simulink model "my_dspsdadc_fixpt"  (Simulink 7.5)
settings: Solver=ode5  SolverMode=SingleTasking  StartTime=0.0  StopTime=.025  FixedStep=1/(512*1024)  MaxStep=1/512000  RelTol=1e-3  AbsTol=1e-6
values from neighbouring files (symbols this model uses):
  Fs = 100000    [bandwidth_chop.m]
undefined symbols (not defined in the file or in its folder): get, sided, Two
libraries: simulink x42, dspsigops x6, dspsnks4 x2, dsparch4 x1, dspmlti4 x1, dspmisc x1
settings Model: Creator=The MathWorks Inc.  LastModifiedBy=Ben  ExtModeTrigMode=oneshot  ExtModeArmWhenConnect=off  ExtModeAutoUpdateStatusClock=off
settings DataIOCC: LimitDataPoints=off  SaveOutput=off  SaveTime=off  SignalLoggingName=logsOut
settings OptimizationCC: BlockReduction=off  BooleanDataType=off  InlineInvariantSignals=on  RollThreshold=2  InitFltsAndDblsToZero=on  EfficientMapNaN2IntZero=off
settings DebuggingCC: SaveWithParameterizedLinksMsg=none  SignalResolutionControl=TryResolveAllWithWarning  SolverPrmCheckMsg=none  MultiTaskDSMMsg=warning  MultiTaskCondExecSysMsg=none  IntegerOverflowMsg=none  ParameterPrecisionLossMsg=none  StrictBusMsg=None  LoggingUnavailableSignals=none
settings HardwareCC: TargetUnknown=on
settings RTWCC: IncludeERTFirstTime=on
settings GRTTargetCC: TargetFcnLib=ansi_tfl_tmw.mat

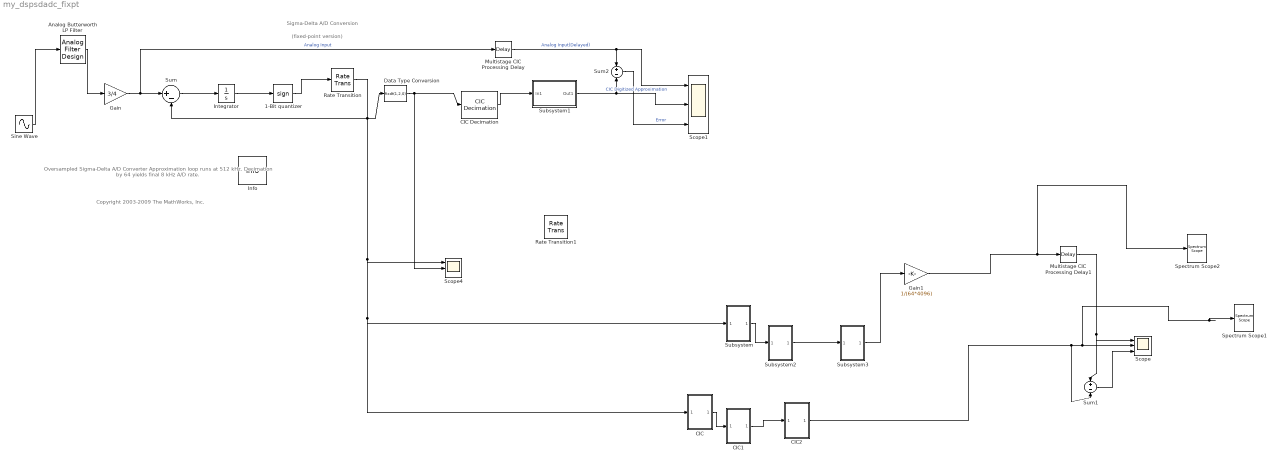
== system my_dspsdadc_fixpt ==
  note: Oversampled Sigma-Delta A/D Converter
      | Approximation loop runs at 512 kHz.
      | Decimation by 64 yields final 8 kHz A/D rate.
  note: Sigma-Delta A/D Conversion
  note: (fixed-point version)
  note: Copyright 2003-2009 The MathWorks, Inc.
  1-Bit quantizer : Signum
  Analog Butterworth LP Filter : dsparch4/Analog Filter Design  method=Butterworth  filttype=Lowpass  N=5  Wlo=2*pi*400  Whi=80  Rp=2  Rs=40
  CIC : Subsystem
  CIC Decimation : dspmlti4/CIC Decimation  DialogController=dspdialog.CICDecimation  filtFrom=Dialog  filtobj=Hm_decim  ftype=Decimator  R=64  M=1  N=5  filterInternals=Full precision  BPS=[32 30 24 20 16 16 16 16 16 16]  FLPS=0  outputWordLength=16  outputFracLength=0  launchFVT=off  framing=Maintain input frame rate
  CIC1 : Subsystem
  CIC2 : Subsystem
  Data Type Conversion : DataTypeConversion  OutDataTypeMode=Specify via dialog  OutDataType=fixdt(1,2,0)  OutDataTypeStr=fixdt(1,2,0)
  Gain : Gain  Gain=3/4  ParameterDataType=sfix(16)  ParameterScaling=2^0  OutDataType=sfix(16)  OutScaling=2^0  SaturateOnIntegerOverflow=on  OutDataTypeStr=Inherit: Same as input  ParamDataTypeStr=Inherit: Same as input
  Gain1 : Gain  Gain=1/(64*4096)  ParameterDataType=sfix(16)  ParameterScaling=2^0  OutDataType=sfix(16)  OutScaling=2^0  SaturateOnIntegerOverflow=on  OutDataTypeStr=Inherit: Same as input  ParamDataTypeStr=Inherit: Same as input
  Info : dspmisc/Info  SystemSampleTime=-1
  Integrator : Integrator
  Multistage CIC Processing Delay : TransportDelay  DelayTime=250/512000
  Multistage CIC Processing Delay1 : TransportDelay  DelayTime=1/10100
  Rate Transition : RateTransition  OutPortSampleTime=1/(512*1024)
  Rate Transition1 : RateTransition  OutPortSampleTime=1/(512*1024)
  Scope : Scope  NumInputPorts=3
      settings: YMin=-5~-5~-5  YMax=5~5~5
  Scope1 : Scope  NumInputPorts=3
      settings: TimeRange=0.025  YMin=-1.1~-1.1~-0.25  YMax=1.1~1.1~0.25  MaxDataPoints=15000
  Scope4 : Scope  NumInputPorts=3
      settings: YMin=-5~-5~-5  YMax=5~5~5  SaveName=ScopeData4
  Sine Wave : Sin  SineType=Sample based  Amplitude=1  Bias=0  Frequency=1  Phase=0  Samples=10000  SampleTime=1/(512*1024)  Offset=0
  Spectrum Scope1 : dspsnks4/Spectrum Scope  DialogController=dspdialog.SpectrumScope  DialogControllerArgs=DataTag1  SystemSampleTime=-1  ScopeProperties=on  Domain=Frequency  HorizSpan=1  UseBuffer=on  BufferSize=128  Overlap=64  inpFftLenInherit=off  FFTlength=4096  numAvg=2  DisplayProperties=off  AxisGrid=on  Memory=off  FrameNumber=on  AxisLegend=off  AxisZoom=off  OpenScopeAtSimStart=on  OpenScopeImmediately=off  FigPos=get(0,'defaultfigureposition')  AxisProperties=off  XUnits=Hertz  XRange=Two-sided ((-Fs/2...Fs/2])  XDisplay=0  InheritXIncr=on  XIncr=1.0  XLabel=Samples  XLimit=Auto  YUnits=dBW/Hertz  XMax=1  XMin=0  YLabel=Magnitude-squared, dB  LineProperties=off  wintypeSpecScope=Hann  RsSpecScope=50  betaSpecScope=5  winsampSpecScope=Periodic  XAxisParamsVer=6.9
      settings: YMin=-100  YMax=100
  Spectrum Scope2 : dspsnks4/Spectrum Scope  DialogController=dspdialog.SpectrumScope  DialogControllerArgs=DataTag2  SystemSampleTime=-1  ScopeProperties=on  Domain=Frequency  HorizSpan=1  UseBuffer=on  BufferSize=128  Overlap=64  inpFftLenInherit=off  FFTlength=4096  numAvg=2  DisplayProperties=off  AxisGrid=on  Memory=off  FrameNumber=on  AxisLegend=off  AxisZoom=off  OpenScopeAtSimStart=on  OpenScopeImmediately=off  FigPos=get(0,'defaultfigureposition')  AxisProperties=off  XUnits=Hertz  XRange=Two-sided ((-Fs/2...Fs/2])  XDisplay=0  InheritXIncr=on  XIncr=1.0  XLabel=Samples  XLimit=Auto  YUnits=dBW/Hertz  XMax=1  XMin=0  YLabel=Magnitude-squared, dB  LineProperties=off  wintypeSpecScope=Hann  RsSpecScope=50  betaSpecScope=5  winsampSpecScope=Periodic  XAxisParamsVer=6.9
      settings: YMin=-100  YMax=100
  Subsystem : Subsystem
  Subsystem1 : Subsystem
      mask Display: disp('Rescaling for\nComparison')
  Subsystem2 : Subsystem
  Subsystem3 : Subsystem
  Sum : Sum  Inputs=|+-  OutDataType=sfix(16)  OutScaling=2^0  SaturateOnIntegerOverflow=on  InputSameDT=on  OutDataTypeStr=Inherit: Same as first input
  Sum1 : Sum  Inputs=+-  OutDataType=sfix(16)  OutScaling=2^0  RndMeth=Nearest  SaturateOnIntegerOverflow=on
  Sum2 : Sum  Inputs=+-  OutDataType=sfix(16)  OutScaling=2^0  RndMeth=Nearest  SaturateOnIntegerOverflow=on
  wires:
  1-Bit quantizer/1 -> Rate Transition/1
  Sum/1 -> Integrator/1
  Gain/1 -> Sum/1, Multistage CIC Processing Delay/1  "Analog Input"
  Data Type Conversion/1 -> Scope4/2, CIC Decimation/1
  CIC Decimation/1 -> Subsystem1/1(In1)
  Sum2/1 -> Scope1/3  "Error"
  Multistage CIC Processing Delay/1 -> Sum2/1, Scope1/1  "Analog Input(Delayed)"
  Subsystem1/1(Out1) -> Sum2/2, Scope1/2  "CIC Digitized Approximation"
  Rate Transition/1 -> Data Type Conversion/1, Sum/2, Scope4/1, Subsystem/1(In1), CIC/1(In1)
  Sine Wave/1 -> Analog Butterworth LP Filter/1
  Analog Butterworth LP Filter/1 -> Gain/1
  Integrator/1 -> 1-Bit quantizer/1
  Subsystem/1(Out1) -> Subsystem2/1(In1)
  Subsystem2/1(Out1) -> Subsystem3/1(In1)
  CIC/1(Out1) -> CIC1/1(In1)
  CIC1/1(Out1) -> CIC2/1(In1)
  CIC2/1(Out1) -> Sum1/2, Scope/2, Spectrum Scope1/1
  Subsystem3/1(Out1) -> Gain1/1
  Sum1/1 -> Scope/3
  Multistage CIC Processing Delay1/1 -> Sum1/1, Scope/1
  Gain1/1 -> Multistage CIC Processing Delay1/1, Spectrum Scope2/1

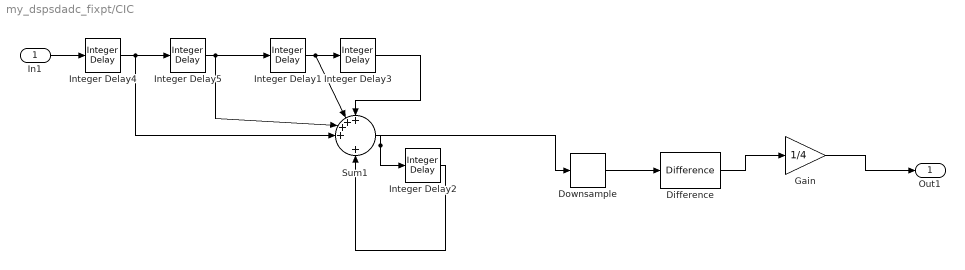
== system my_dspsdadc_fixpt/CIC ==
  In1 : Inport
  Difference : simulink/Discrete/Difference  SystemSampleTime=-1  ICPrevInput=0.0  OutMin=[]  OutMax=[]  OutDataType=fixdt(1, 16)  OutScaling=2^-10  DoSatur=off
  Downsample : dspsigops/Downsample  N=4  phase=0  ic=0  smode=Allow multirate  fmode=Maintain input frame size
  Gain : Gain  Gain=1/4  ParameterDataType=sfix(16)  ParameterScaling=2^0  OutDataType=sfix(16)  OutScaling=2^0  SaturateOnIntegerOverflow=on  OutDataTypeStr=Inherit: Same as input  ParamDataTypeStr=Inherit: Same as input
  Integer Delay{1..5} (5 alike) : simulink/Discrete/Integer Delay  vinit=0.0  samptime=-1  NumDelays=1
  Sum1 : Sum  Inputs=++++||+  OutDataType=sfix(16)  OutScaling=2^0  SaturateOnIntegerOverflow=on  InputSameDT=on  OutDataTypeStr=Inherit: Same as first input
  Out1 : Outport
  wires:
  Integer Delay4/1 -> Integer Delay5/1, Sum1/4
  Integer Delay5/1 -> Integer Delay1/1, Sum1/3
  Sum1/1 -> Downsample/1, Integer Delay2/1
  Downsample/1 -> Difference/1
  Integer Delay2/1 -> Sum1/5
  Integer Delay1/1 -> Integer Delay3/1, Sum1/2
  Integer Delay3/1 -> Sum1/1
  In1/1 -> Integer Delay4/1
  Difference/1 -> Gain/1
  Gain/1 -> Out1/1

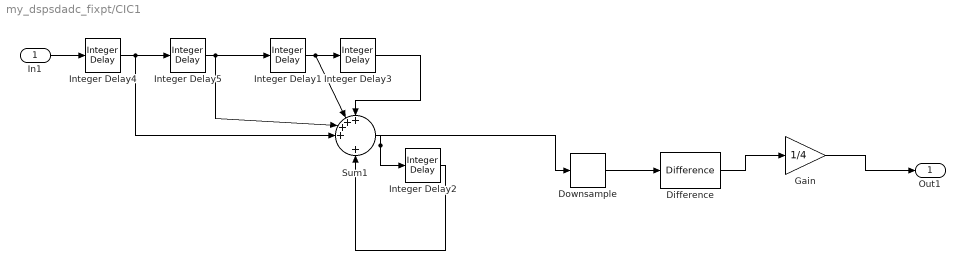
== system my_dspsdadc_fixpt/CIC1 ==
  In1 : Inport
  Difference : simulink/Discrete/Difference  SystemSampleTime=-1  ICPrevInput=0.0  OutMin=[]  OutMax=[]  OutDataType=fixdt(1, 16)  OutScaling=2^-10  DoSatur=off
  Downsample : dspsigops/Downsample  N=4  phase=0  ic=0  smode=Allow multirate  fmode=Maintain input frame size
  Gain : Gain  Gain=1/4  ParameterDataType=sfix(16)  ParameterScaling=2^0  OutDataType=sfix(16)  OutScaling=2^0  SaturateOnIntegerOverflow=on  OutDataTypeStr=Inherit: Same as input  ParamDataTypeStr=Inherit: Same as input
  Integer Delay{1..5} (5 alike) : simulink/Discrete/Integer Delay  vinit=0.0  samptime=-1  NumDelays=1
  Sum1 : Sum  Inputs=++++||+  OutDataType=sfix(16)  OutScaling=2^0  SaturateOnIntegerOverflow=on  InputSameDT=on  OutDataTypeStr=Inherit: Same as first input
  Out1 : Outport
  wires:
  Integer Delay4/1 -> Integer Delay5/1, Sum1/4
  Integer Delay5/1 -> Integer Delay1/1, Sum1/3
  Sum1/1 -> Downsample/1, Integer Delay2/1
  Downsample/1 -> Difference/1
  Integer Delay2/1 -> Sum1/5
  Integer Delay1/1 -> Integer Delay3/1, Sum1/2
  Integer Delay3/1 -> Sum1/1
  In1/1 -> Integer Delay4/1
  Difference/1 -> Gain/1
  Gain/1 -> Out1/1

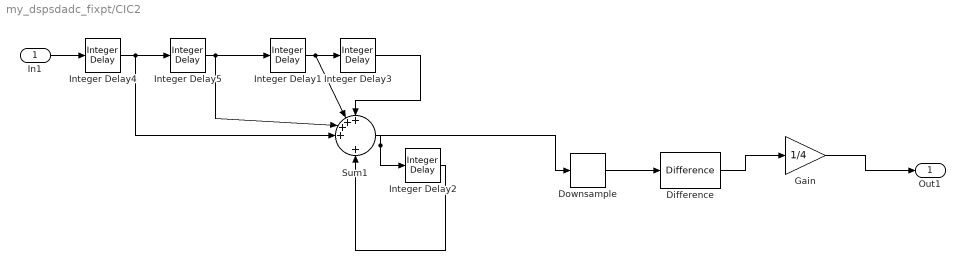
== system my_dspsdadc_fixpt/CIC2 ==
  In1 : Inport
  Difference : simulink/Discrete/Difference  SystemSampleTime=-1  ICPrevInput=0.0  OutMin=[]  OutMax=[]  OutDataType=fixdt(1, 16)  OutScaling=2^-10  DoSatur=off
  Downsample : dspsigops/Downsample  N=4  phase=0  ic=0  smode=Allow multirate  fmode=Maintain input frame size
  Gain : Gain  Gain=1/4  ParameterDataType=sfix(16)  ParameterScaling=2^0  OutDataType=sfix(16)  OutScaling=2^0  SaturateOnIntegerOverflow=on  OutDataTypeStr=Inherit: Same as input  ParamDataTypeStr=Inherit: Same as input
  Integer Delay{1..5} (5 alike) : simulink/Discrete/Integer Delay  vinit=0.0  samptime=-1  NumDelays=1
  Sum1 : Sum  Inputs=++++||+  OutDataType=sfix(16)  OutScaling=2^0  SaturateOnIntegerOverflow=on  InputSameDT=on  OutDataTypeStr=Inherit: Same as first input
  Out1 : Outport
  wires:
  Integer Delay4/1 -> Integer Delay5/1, Sum1/4
  Integer Delay5/1 -> Integer Delay1/1, Sum1/3
  Sum1/1 -> Downsample/1, Integer Delay2/1
  Downsample/1 -> Difference/1
  Integer Delay2/1 -> Sum1/5
  Integer Delay1/1 -> Integer Delay3/1, Sum1/2
  Integer Delay3/1 -> Sum1/1
  In1/1 -> Integer Delay4/1
  Difference/1 -> Gain/1
  Gain/1 -> Out1/1

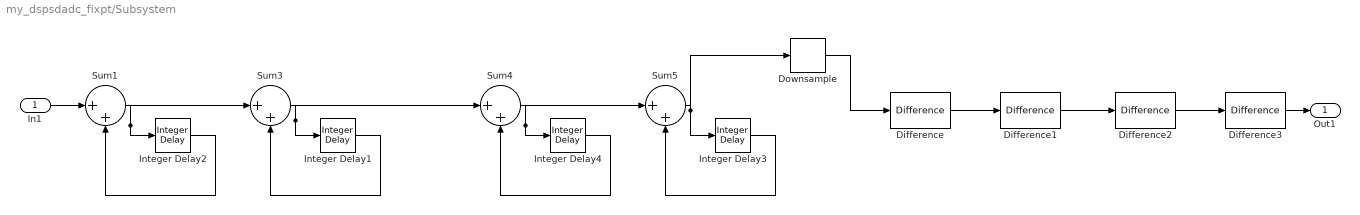
== system my_dspsdadc_fixpt/Subsystem ==
  In1 : Inport
  Difference{,1..3} (4 alike) : simulink/Discrete/Difference  SystemSampleTime=-1  ICPrevInput=0.0  OutMin=[]  OutMax=[]  OutDataType=fixdt(1, 16)  OutScaling=2^-10  DoSatur=off
  Downsample : dspsigops/Downsample  N=4  phase=0  ic=0  smode=Allow multirate  fmode=Maintain input frame size
  Integer Delay{1..4} (4 alike) : simulink/Discrete/Integer Delay  vinit=0.0  samptime=-1  NumDelays=1
  Sum{1,3..5} (4 alike) : Sum  Inputs=|++  OutDataType=sfix(16)  OutScaling=2^0  SaturateOnIntegerOverflow=on  InputSameDT=on  OutDataTypeStr=Inherit: Same as first input
  Out1 : Outport
  wires:
  Sum1/1 -> Integer Delay2/1, Sum3/1
  Integer Delay2/1 -> Sum1/2
  Sum3/1 -> Integer Delay1/1, Sum4/1
  Integer Delay1/1 -> Sum3/2
  Sum4/1 -> Integer Delay4/1, Sum5/1
  Integer Delay4/1 -> Sum4/2
  Sum5/1 -> Integer Delay3/1, Downsample/1
  Integer Delay3/1 -> Sum5/2
  Difference/1 -> Difference1/1
  Difference1/1 -> Difference2/1
  Difference2/1 -> Difference3/1
  Downsample/1 -> Difference/1
  In1/1 -> Sum1/1
  Difference3/1 -> Out1/1

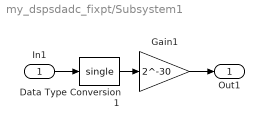
== system my_dspsdadc_fixpt/Subsystem1 ==
  In1 : Inport  OutDataType=sfix(16)  OutScaling=2^0
  Data Type Conversion1 : DataTypeConversion  OutDataTypeMode=single  OutDataType=sfix(2)  OutScaling=2^0  OutDataTypeStr=single
  Gain1 : Gain  Gain=2^-30  ParameterDataType=sfix(16)  ParameterScaling=2^0  OutDataType=sfix(16)  OutScaling=2^0  SaturateOnIntegerOverflow=on  OutDataTypeStr=Inherit: Same as input  ParamDataTypeStr=Inherit: Same as input
  Out1 : Outport  OutDataType=sfix(16)  OutScaling=2^0
  wires:
  Data Type Conversion1/1 -> Gain1/1
  In1/1 -> Data Type Conversion1/1
  Gain1/1 -> Out1/1

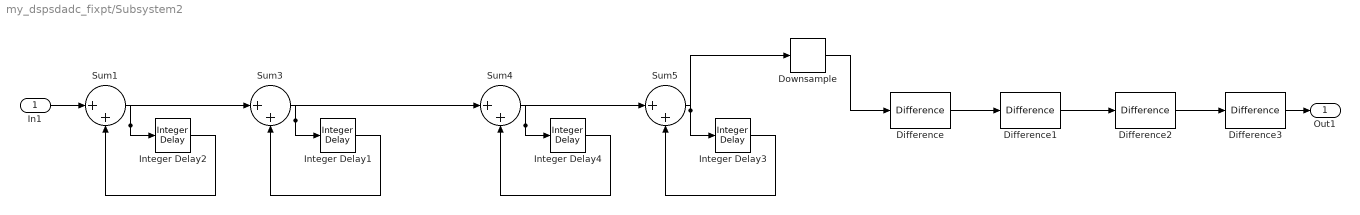
== system my_dspsdadc_fixpt/Subsystem2 ==
  In1 : Inport
  Difference{,1..3} (4 alike) : simulink/Discrete/Difference  SystemSampleTime=-1  ICPrevInput=0.0  OutMin=[]  OutMax=[]  OutDataType=fixdt(1, 16)  OutScaling=2^-10  DoSatur=off
  Downsample : dspsigops/Downsample  N=4  phase=0  ic=0  smode=Allow multirate  fmode=Maintain input frame size
  Integer Delay{1..4} (4 alike) : simulink/Discrete/Integer Delay  vinit=0.0  samptime=-1  NumDelays=1
  Sum{1,3..5} (4 alike) : Sum  Inputs=|++  OutDataType=sfix(16)  OutScaling=2^0  SaturateOnIntegerOverflow=on  InputSameDT=on  OutDataTypeStr=Inherit: Same as first input
  Out1 : Outport
  wires:
  Sum1/1 -> Integer Delay2/1, Sum3/1
  Integer Delay2/1 -> Sum1/2
  Sum3/1 -> Integer Delay1/1, Sum4/1
  Integer Delay1/1 -> Sum3/2
  Sum4/1 -> Integer Delay4/1, Sum5/1
  Integer Delay4/1 -> Sum4/2
  Sum5/1 -> Integer Delay3/1, Downsample/1
  Integer Delay3/1 -> Sum5/2
  Difference/1 -> Difference1/1
  Difference1/1 -> Difference2/1
  Difference2/1 -> Difference3/1
  Downsample/1 -> Difference/1
  In1/1 -> Sum1/1
  Difference3/1 -> Out1/1

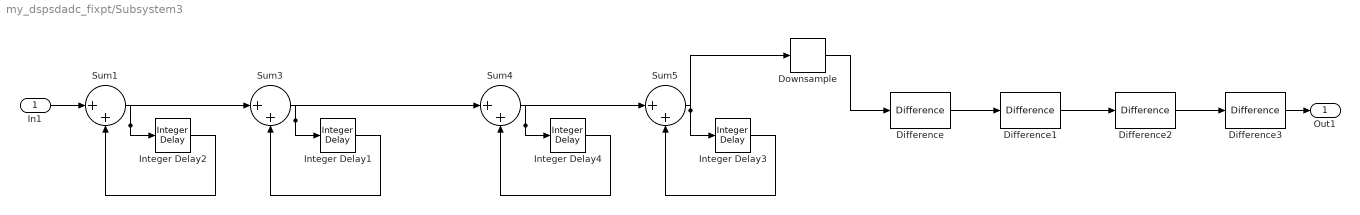
== system my_dspsdadc_fixpt/Subsystem3 ==
  In1 : Inport
  Difference{,1..3} (4 alike) : simulink/Discrete/Difference  SystemSampleTime=-1  ICPrevInput=0.0  OutMin=[]  OutMax=[]  OutDataType=fixdt(1, 16)  OutScaling=2^-10  DoSatur=off
  Downsample : dspsigops/Downsample  N=4  phase=0  ic=0  smode=Allow multirate  fmode=Maintain input frame size
  Integer Delay{1..4} (4 alike) : simulink/Discrete/Integer Delay  vinit=0.0  samptime=-1  NumDelays=1
  Sum{1,3..5} (4 alike) : Sum  Inputs=|++  OutDataType=sfix(16)  OutScaling=2^0  SaturateOnIntegerOverflow=on  InputSameDT=on  OutDataTypeStr=Inherit: Same as first input
  Out1 : Outport
  wires:
  Sum1/1 -> Integer Delay2/1, Sum3/1
  Integer Delay2/1 -> Sum1/2
  Sum3/1 -> Integer Delay1/1, Sum4/1
  Integer Delay1/1 -> Sum3/2
  Sum4/1 -> Integer Delay4/1, Sum5/1
  Integer Delay4/1 -> Sum4/2
  Sum5/1 -> Integer Delay3/1, Downsample/1
  Integer Delay3/1 -> Sum5/2
  Difference/1 -> Difference1/1
  Difference1/1 -> Difference2/1
  Difference2/1 -> Difference3/1
  Downsample/1 -> Difference/1
  In1/1 -> Sum1/1
  Difference3/1 -> Out1/1
